simulink model "float_sch_SNEO"  (R2020a)
settings: Solver=VariableStepAuto  StartTime=0  StopTime=180  RelTol=1e-3
values from neighbouring files (symbols this model uses):
  feature_buffer = fs    (= 30000)    [float_sch_run_SNEO.m]
  feature_gain = [1]    [float_sch_run_SNEO.m]
  fs = 30000    [float_sch_run_SNEO.m]
  refractory = 10^-3    (= 0.001)    [float_sch_run_SNEO.m]
  TEO_buffer = w_smooth    (= 30)    [float_sch_run_SNEO.m]
  w_smooth = fs/1000    (= 30)    [float_sch_run_SNEO.m]
libraries: dspfdesign x2, dspsigops x1, dspswit3 x1, dspstat3 x1, simulink x1, hdlsllib x1
settings Model: SimulationMode=rapid-accelerator  Creator=diflo  LastModifiedBy=diflo

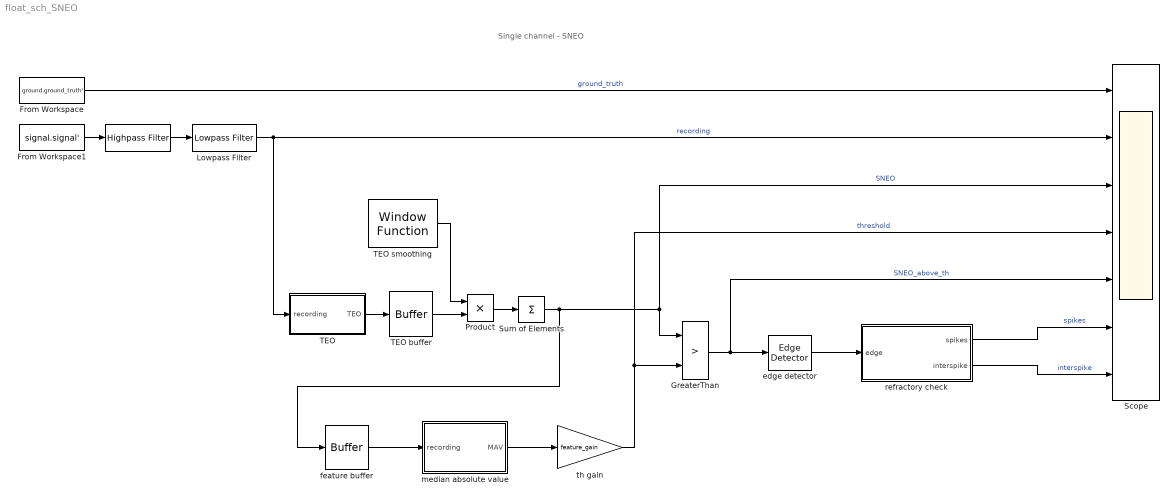
== system float_sch_SNEO ==
  note: Single channel - SNEO
  " " : dspfdesign/Highpass Filter  FilterType=IIR  DesignForMinimumOrder=on  FilterOrder=50  StopbandFrequency=1  PassbandFrequency=300  StopbandAttenuation=80  PassbandRipple=0.1  InheritSampleRate=off  SampleRate=fs  SimulateUsing=Interpreted execution  roundingMode=Floor  coeffsDataTypeStr=fixdt(1,16)
  From Workspace : FromWorkspace  VariableName=ground.ground_truth'  SampleTime=1/fs
  From Workspace1 : FromWorkspace  VariableName=signal.signal'  SampleTime=1/fs
  GreaterThan : RelationalOperator  Operator=>  OutDataTypeStr=boolean  RndMeth=Simplest
  Lowpass Filter : dspfdesign/Lowpass Filter  FilterType=IIR  DesignForMinimumOrder=on  FilterOrder=3  PassbandFrequency=3500  StopbandFrequency=8500  PassbandRipple=0.1  StopbandAttenuation=80  InheritSampleRate=off  SampleRate=fs  SimulateUsing=Interpreted execution  roundingMode=Floor  coeffsDataTypeStr=fixdt(1,16)
  Product : Product
  Scope : Scope  NumInputPorts=7
  Sum of Elements : Sum  Inputs=+
  TEO : Subsystem
  TEO buffer : Buffer  N=TEO_buffer  V=TEO_buffer_overlap  OutputFrames=off
  TEO smoothing : dspsigops/Window Function  winmode=Generate window  wintype=Hamming  sampmode=Discrete  samptime=1/fs  N=w_smooth  Rs=50  beta=10  winsamp=Symmetric  UserWindow=hamming  OptParams=off  UserParams={'symmetric'}  dataType=double  isSigned=on  wordLen=16  udDataType=sfix(16)  fracBitsMode=Best precision  numFracBits=15  roundingMode=Floor  overflowMode=off  numSidelobes=4  sidelobeLevel=-30
      settings: SourceProductBaseCode=DS
  edge detector : dspswit3/Edge Detector  InputProcessing=Columns as channels (frame based)
      settings: SourceProductBaseCode=DS
  feature buffer : Buffer  N=feature_buffer  OutputFrames=off
  median absolute value : Subsystem
  refractory check : Subsystem
  th gain : Gain  Gain=feature_gain
  wires:
  TEO smoothing/1 -> Product/1
  TEO buffer/1 -> Product/2
  Product/1 -> Sum of Elements/1
  TEO/1(TEO) -> TEO buffer/1
  median absolute value/1(MAV) -> th gain/1
  feature buffer/1 -> median absolute value/1(recording)
  Sum of Elements/1 -> Scope/3, GreaterThan/1, feature buffer/1  "SNEO"
  th gain/1 -> GreaterThan/2, Scope/4  "threshold"
  GreaterThan/1 -> Scope/5, edge detector/1  "SNEO_above_th"
  edge detector/1 -> refractory check/1("  edge")
  refractory check/1(" spikes") -> Scope/6  "spikes"
  refractory check/2(interspike) -> Scope/7  "interspike"
  From Workspace/1 -> Scope/1  "ground_truth"
  From Workspace1/1 -> " "/1
  " "/1 -> Lowpass Filter/1
  Lowpass Filter/1 -> Scope/2, TEO/1(recording)  "recording"

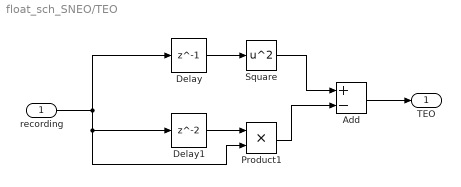
== system float_sch_SNEO/TEO ==
  recording : Inport
  Add : Sum  Inputs=+-
  Delay : Delay  DelayLength=1  InitialCondition=0  SampleTime=1/30000
  Delay1 : Delay  InitialCondition=0  SampleTime=1/30000
  Product1 : Product
  Square : Math  Operator=square  SaturateOnIntegerOverflow=on
  TEO : Outport
  wires:
  Delay1/1 -> Product1/1
  Square/1 -> Add/1
  Add/1 -> TEO/1
  Delay/1 -> Square/1
  Product1/1 -> Add/2
  recording/1 -> Delay/1, Delay1/1, Product1/2

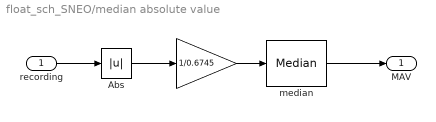
== system float_sch_SNEO/median absolute value ==
  recording : Inport
  "  " : Gain  Gain=1/0.6745
  Abs : Abs
  median : dspstat3/Median  sortAlg=Quick sort  directionMode=Each column  dimension=1  roundingMode=Floor  overflowMode=off  accumDataTypeStr=Inherit: Same as product output  accumLastDataTypeStr=Inherit: Same as product output  outputDataTypeStr=Inherit: Same as accumulator  outputMin=[]  outputMax=[]  outputLastDataTypeStr=Inherit: Same as accumulator
      settings: SourceProductBaseCode=DS  allowOverrides=off
  MAV : Outport
  wires:
  Abs/1 -> "  "/1
  "  "/1 -> median/1
  recording/1 -> Abs/1
  median/1 -> MAV/1

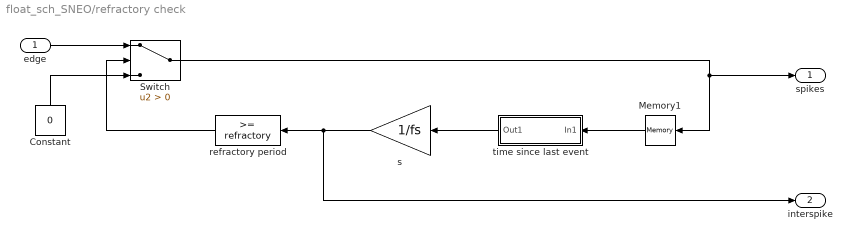
== system float_sch_SNEO/refractory check ==
  "  edge" : Inport
  Constant : Constant  Value=0
  Memory1 : Memory  InheritSampleTime=on
  Switch : Switch  Criteria=u2 > Threshold
  refractory period : simulink/Logic and Bit Operations/Compare To Constant  relop=>=  const=refractory  OutDataTypeStr=boolean
  s : Gain  Gain=1/fs  ParamDataTypeStr=double
  time since last event : Subsystem
  " spikes" : Outport
  interspike : Outport  Port=2
  wires:
  "  edge"/1 -> Switch/1
  Memory1/1 -> time since last event/1(In1)
  time since last event/1(Out1) -> s/1
  Constant/1 -> Switch/3
  s/1 -> refractory period/1, interspike/1
  Switch/1 -> " spikes"/1, Memory1/1
  refractory period/1 -> Switch/2

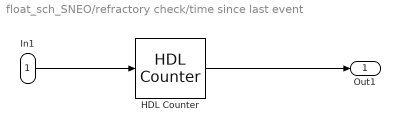
== system float_sch_SNEO/refractory check/time since last event ==
  In1 : Inport
  HDL Counter : hdlsllib/Sources/HDL Counter  CountType=Free running  CountInit=1  CountStep=1  CountMax=25  CountFromType=Initial value  CountFrom=1  CountResetPort=on  CountLoadPort=off  CountEnbPort=off  CountDirPort=off  CountDataType=Unsigned  CountWordLen=32  CountFracLen=0  CountSampTime=1
  Out1 : Outport
  wires:
  In1/1 -> HDL Counter/1
  HDL Counter/1 -> Out1/1
